simulink model "gps_sim_navtoolbox"  (R2024b)
settings: Solver=VariableStepAuto  StartTime=0.0  StopTime=25  RelTol=1e-3
undefined symbols (not defined in the file or in its folder): altitude, latitude, longitude, service, status
libraries: ros2lib x5, sensorgpslib x4
settings Model: LastModifiedBy=DCHOME

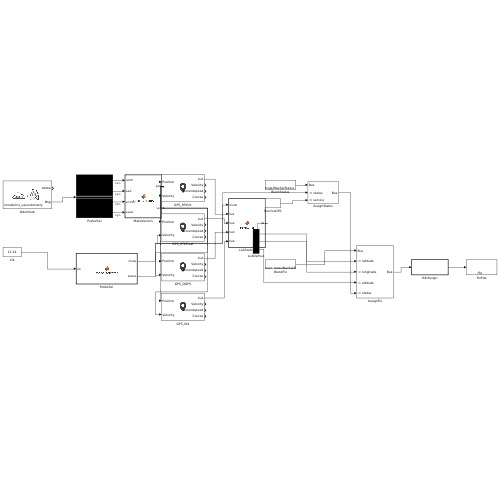
[thumbnail: Simulink's stored preview of the top-level diagram]
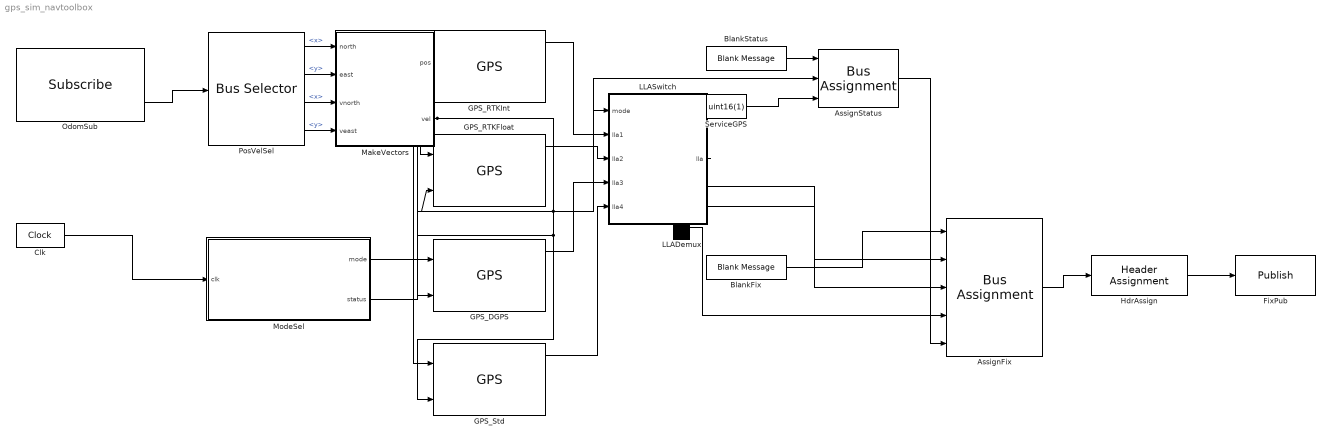
== system gps_sim_navtoolbox ==
  AssignFix : BusAssignment  AssignedSignals=latitude,longitude,altitude,status
  AssignStatus : BusAssignment  AssignedSignals=status,service
  BlankFix : ros2lib/Blank Message  messageClass=Message  entityType=sensor_msgs/NavSatFix  messageType=sensor_msgs/NavSatFix  SampleTime=inf
  BlankStatus : ros2lib/Blank Message  messageClass=Message  entityType=sensor_msgs/NavSatStatus  messageType=sensor_msgs/NavSatStatus  SampleTime=inf
  Clk : DigitalClock  SampleTime=0.2
  FixPub : ros2lib/Publish  topicSource=Select from ROS network  topic=/fix  messageType=sensor_msgs/NavSatFix  QOSHistory=Keep last  QOSDepth=1  QOSReliability=Reliable  QOSDurability=Volatile  QOSDeadline=Inf  QOSLifespan=Inf  QOSLiveliness=Automatic  QOSLeaseDuration=Inf  QOSAvoidROSNamespaceConventions=off
  GPS_DGPS : sensorgpslib/GPS  DispRefFrame=NED  PositionInputFormat=Local  ReferenceLocation=[-35.363262 149.165237 0]  HorizontalPositionAccuracy=0.4  VerticalPositionAccuracy=0.6  VelocityAccuracy=0.2  DecayFactor=0.999  SeedDouble=67  SimulateUsing=Interpreted execution
  GPS_RTKFloat : sensorgpslib/GPS  DispRefFrame=NED  PositionInputFormat=Local  ReferenceLocation=[-35.363262 149.165237 0]  HorizontalPositionAccuracy=0.05  VerticalPositionAccuracy=0.08  VelocityAccuracy=0.05  DecayFactor=0.999  SeedDouble=67  SimulateUsing=Interpreted execution
  GPS_RTKInt : sensorgpslib/GPS  DispRefFrame=NED  PositionInputFormat=Local  ReferenceLocation=[-35.363262 149.165237 0]  HorizontalPositionAccuracy=0.01  VerticalPositionAccuracy=0.02  VelocityAccuracy=0.02  DecayFactor=0.999  SeedDouble=67  SimulateUsing=Interpreted execution
  GPS_Std : sensorgpslib/GPS  DispRefFrame=NED  PositionInputFormat=Local  ReferenceLocation=[-35.363262 149.165237 0]  HorizontalPositionAccuracy=1.5  VerticalPositionAccuracy=3  VelocityAccuracy=0.5  DecayFactor=0.999  SeedDouble=67  SimulateUsing=Interpreted execution
  HdrAssign : ros2lib/Header Assignment  SetFrameID=on  FrameID=gps  InsertTimeStamp=on  SetHeaderFieldName=Use the default header field name  HeaderFieldName=header
  LLADemux : Demux  Outputs=3
  LLASwitch : MATLAB Function  TreatAsAtomicUnit=on
  MakeVectors : MATLAB Function  TreatAsAtomicUnit=on
  ModeSel : MATLAB Function  TreatAsAtomicUnit=on
  OdomSub : ros2lib/Subscribe  topicSource=Specify your own  topic=/model/iris_uav/odometry  messageType=nav_msgs/Odometry  sampleTime=0.2  QOSHistory=Keep last  QOSDepth=1  QOSReliability=Reliable  QOSDurability=Volatile  QOSDeadline=Inf  QOSLifespan=Inf  QOSLiveliness=Automatic  QOSLeaseDuration=Inf  QOSAvoidROSNamespaceConventions=off
  PosVelSel : BusSelector  OutputSignals=pose.pose.position.x,pose.pose.position.y,twist.twist.linear.x,twist.twist.linear.y
  ServiceGPS : Constant  Value=uint16(1)
  wires:
  OdomSub/2 -> PosVelSel/1
  PosVelSel/1 -> MakeVectors/1(north)  "<x>"
  PosVelSel/2 -> MakeVectors/2(east)  "<y>"
  PosVelSel/3 -> MakeVectors/3(vnorth)  "<x>"
  PosVelSel/4 -> MakeVectors/4(veast)  "<y>"
  Clk/1 -> ModeSel/1(clk)
  MakeVectors/1(pos) -> GPS_RTKInt/1, GPS_RTKFloat/1, GPS_DGPS/1, GPS_Std/1
  MakeVectors/2(vel) -> GPS_DGPS/2, GPS_Std/2, GPS_RTKFloat/2, GPS_RTKInt/2
  GPS_RTKInt/1 -> LLASwitch/2(lla1)
  GPS_RTKFloat/1 -> LLASwitch/3(lla2)
  GPS_DGPS/1 -> LLASwitch/4(lla3)
  GPS_Std/1 -> LLASwitch/5(lla4)
  ModeSel/1(mode) -> LLASwitch/1(mode)
  BlankStatus/1 -> AssignStatus/1
  ModeSel/2(status) -> AssignStatus/2
  ServiceGPS/1 -> AssignStatus/3
  LLASwitch/1(lla) -> LLADemux/1
  BlankFix/1 -> AssignFix/1
  LLADemux/1 -> AssignFix/2
  LLADemux/2 -> AssignFix/3
  LLADemux/3 -> AssignFix/4
  AssignStatus/1 -> AssignFix/5
  AssignFix/1 -> HdrAssign/1
  HdrAssign/1 -> FixPub/1

== matlab function gps_sim_navtoolbox/ModeSel ==
  data: clk input; mode output; status output
function [mode, status] = mode_selector(clk)
    persistent state_idx state_until
    if isempty(state_idx)
        state_idx = int32(2);
        state_until = clk + (-8.0 * log(rand()));
    end
    weights = [0.05, 0.70, 0.20, 0.05];
    statuses = int8([2, 2, 1, 0]);
    if clk >= state_until
        idx_others = int32(setdiff([1,2,3,4], double(state_idx)));
        w_others = weights(idx_others);
        total = sum(w_others);
        rr = rand()*total;
        acc = 0; chosen = idx_others(end);
        for k = 1:numel(idx_others)
            acc = acc + w_others(k);
            if rr <= acc
                chosen = idx_others(k);
                break;
            end
        end
        state_idx = chosen;
        state_until = clk + (-8.0 * log(rand()));
    end
    mode = state_idx;
    status = statuses(state_idx);
end

== matlab function gps_sim_navtoolbox/MakeVectors ==
  data: north input; pos output; east input; vnorth input; veast input; vel output
function [pos, vel] = make_vectors(north, east, vnorth, veast)
    pos = [north, east, 0];
    vel = [vnorth, veast, 0];
end

== matlab function gps_sim_navtoolbox/LLASwitch ==
  data: mode input; lla output; lla1 input; lla2 input; lla3 input; lla4 input
function lla = select_lla(mode, lla1, lla2, lla3, lla4)
    switch mode
        case 1
            lla = lla1;
        case 2
            lla = lla2;
        case 3
            lla = lla3;
        otherwise
            lla = lla4;
    end
end
